simulink model "velocity_tracking_2nd_order"  (R2018b)
settings: Solver=ode8  StartTime=0.0  StopTime=14  FixedStep=0.05  RelTol=1e-3
settings Model: Creator=suvo.ganguli  LastModifiedBy=suvo.ganguli

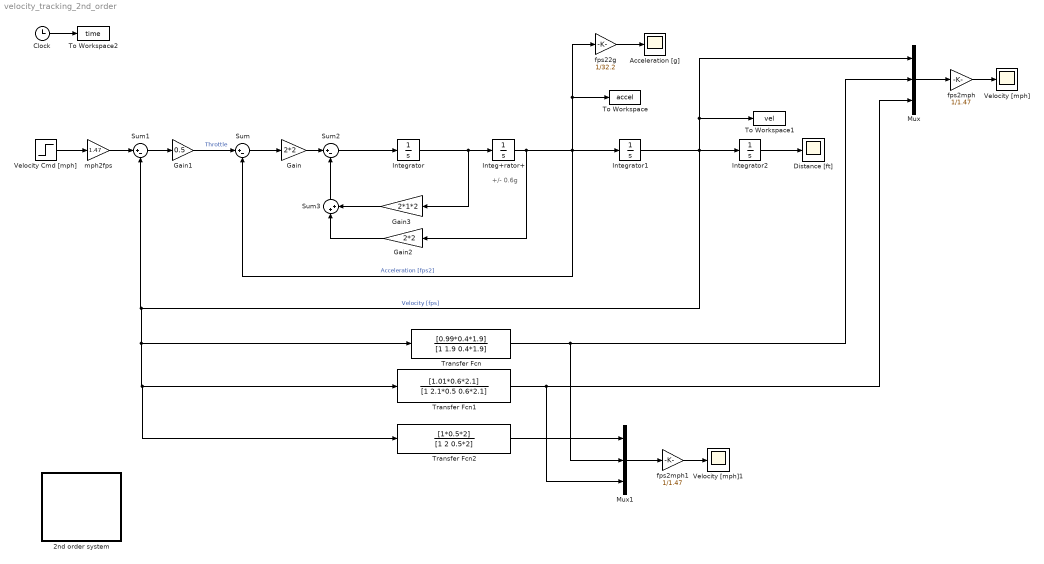
== system velocity_tracking_2nd_order ==
  note: +/- 0.6g
  2nd order system : Subsystem
  Acceleration [g] : Scope
  Clock : Clock
  Distance [ft] : Scope
  Gain : Gain  Gain=2*2
  Gain1 : Gain  Gain=0.5
  Gain2 : Gain  Gain=2*2
  Gain3 : Gain  Gain=2*1*2
  Integ+rator+ : Integrator  LimitOutput=on  UpperSaturationLimit=0.6*32.2  LowerSaturationLimit=-0.6*32.2
  Integrator : Integrator
  Integrator1 : Integrator
  Integrator2 : Integrator
  Mux : Mux  Inputs=3
  Mux1 : Mux  Inputs=3
  Sum : Sum  Inputs=|+-
  Sum1 : Sum  Inputs=|+-
  Sum2 : Sum  Inputs=|+-
  Sum3 : Sum  Inputs=|++
  To Workspace : ToWorkspace  VariableName=accel  SampleTime=-1
  To Workspace1 : ToWorkspace  VariableName=vel  SampleTime=-1
  To Workspace2 : ToWorkspace  VariableName=time  SampleTime=-1
  Transfer Fcn : TransferFcn  Numerator=[0.99*0.4*1.9]  Denominator=[1 1.9 0.4*1.9]
  Transfer Fcn1 : TransferFcn  Numerator=[1.01*0.6*2.1]  Denominator=[1 2.1*0.5 0.6*2.1]
  Transfer Fcn2 : TransferFcn  Numerator=[1*0.5*2]  Denominator=[1 2 0.5*2]
  Velocity [mph] : Scope
  Velocity [mph]1 : Scope
  Velocity Cmd [mph] : Step  Time=0  After=45  SampleTime=0
  fps22g : Gain  Gain=1/32.2
  fps2mph : Gain  Gain=1/1.47
  fps2mph1 : Gain  Gain=1/1.47
  mph2fps : Gain  Gain=1.47
  wires:
  Sum/1 -> Gain/1
  Integ+rator+/1 -> Gain2/1, Integrator1/1, To Workspace/1, fps22g/1, Sum/2  "Acceleration [fps2]"
  Sum1/1 -> Gain1/1
  Integrator1/1 -> Transfer Fcn2/1, Transfer Fcn1/1, Transfer Fcn/1, Sum1/2, Integrator2/1, Mux/1, To Workspace1/1  "Velocity [fps]"
  Gain1/1 -> Sum/1  "Throttle"
  Integrator2/1 -> Distance [ft]/1
  mph2fps/1 -> Sum1/1
  fps2mph/1 -> Velocity [mph]/1
  fps22g/1 -> Acceleration [g]/1
  Velocity Cmd [mph]/1 -> mph2fps/1
  Clock/1 -> To Workspace2/1
  Integrator/1 -> Gain3/1, Integ+rator+/1
  Sum3/1 -> Sum2/2
  Gain/1 -> Sum2/1
  Gain2/1 -> Sum3/1
  Gain3/1 -> Sum3/2
  Sum2/1 -> Integrator/1
  Mux/1 -> fps2mph/1
  Transfer Fcn/1 -> Mux1/2, Mux/2
  Transfer Fcn1/1 -> Mux1/3, Mux/3
  Mux1/1 -> fps2mph1/1
  fps2mph1/1 -> Velocity [mph]1/1
  Transfer Fcn2/1 -> Mux1/1

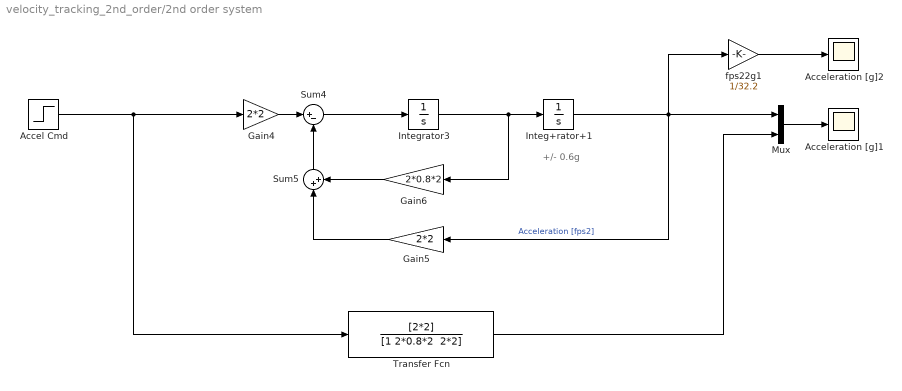
== system velocity_tracking_2nd_order/2nd order system ==
  note: +/- 0.6g
  Accel Cmd : Step  Time=0  Before=20  After=45  SampleTime=0
  Acceleration [g]1 : Scope
  Acceleration [g]2 : Scope
  Gain4 : Gain  Gain=2*2
  Gain5 : Gain  Gain=2*2
  Gain6 : Gain  Gain=2*0.8*2
  Integ+rator+1 : Integrator  LimitOutput=on  UpperSaturationLimit=0.6*32.2*100  LowerSaturationLimit=-0.6*32.2*100
  Integrator3 : Integrator
  Mux : Mux  Inputs=2
  Sum4 : Sum  Inputs=|+-
  Sum5 : Sum  Inputs=|++
  Transfer Fcn : TransferFcn  Numerator=[2*2]  Denominator="[1 2*0.8*2  2*2]"
  fps22g1 : Gain  Gain=1/32.2
  wires:
  Gain4/1 -> Sum4/1
  Transfer Fcn/1 -> Mux/2
  Sum4/1 -> Integrator3/1
  Integrator3/1 -> Integ+rator+1/1, Gain6/1
  fps22g1/1 -> Acceleration [g]2/1
  Accel Cmd/1 -> Transfer Fcn/1, Gain4/1
  Integ+rator+1/1 -> fps22g1/1, Gain5/1, Mux/1  "Acceleration [fps2]"
  Gain5/1 -> Sum5/1
  Gain6/1 -> Sum5/2
  Sum5/1 -> Sum4/2
  Mux/1 -> Acceleration [g]1/1
